simulink model "compared_sim_pizeo"  (R2022b)
settings: Solver=FixedStepAuto  StartTime=0.0  StopTime=5  FixedStep=0.001  RelTol=1e-3  EnableMultiTasking=on
settings Model: Creator=Administrator  LastModifiedBy=huheyu
settings SolverCC: AlgebraicLoopSolver=TrustRegion
settings DataIOCC: LimitDataPoints=on  SaveFormat=Array  ReturnWorkspaceOutputs=off
settings OptimizationCC: LifeSpan=inf
settings DebuggingCC: UnderspecifiedInitializationDetection=Classic  MergeDetectMultiDrivingBlocksExec=none  SolverPrmCheckMsg=warning  UnconnectedInputMsg=warning  UnconnectedOutputMsg=warning  UnconnectedLineMsg=warning  StateNameClashWarn=warning  SFUnexpectedBacktrackingDiag=warning  SFNoUnconditionalDefaultTransitionDiag=warning  SFExecutionAtInitializationDiag=none  ArithmeticOperatorsInVariantConditions=warning
settings HardwareCC: ProdBitPerPointer=32  ProdBitPerSizeT=32  ProdBitPerPtrDiffT=32  ProdLargestAtomicFloat=None  ProdIntDivRoundTo=Undefined  ProdEndianess=Unspecified  ProdWordSize=32  ProdHWDeviceType=32-bit Generic
settings ModelReferenceCC: EnableRefExpFcnMdlSchedulingChecks=on  PropagateSignalLabelsOutOfModel=off
settings SFSimCC: SimUseLocalCustomCode=off  CustomCodeUndefinedFunction=UseInterfaceOnly
settings RTWCC: RTWUseLocalCustomCode=off  DLArmComputeVersion=19.05
settings CodeAppCC: StateflowObjectComments=on
settings GRTTargetCC: TargetLangStandard=C89/C90 (ANSI)
settings ConfigComp: CovMetricSettings=dw  CovSaveCumulativeToWorkspaceVar=on  CovSaveSingleToWorkspaceVar=on  CovExternalEMLEnable=off

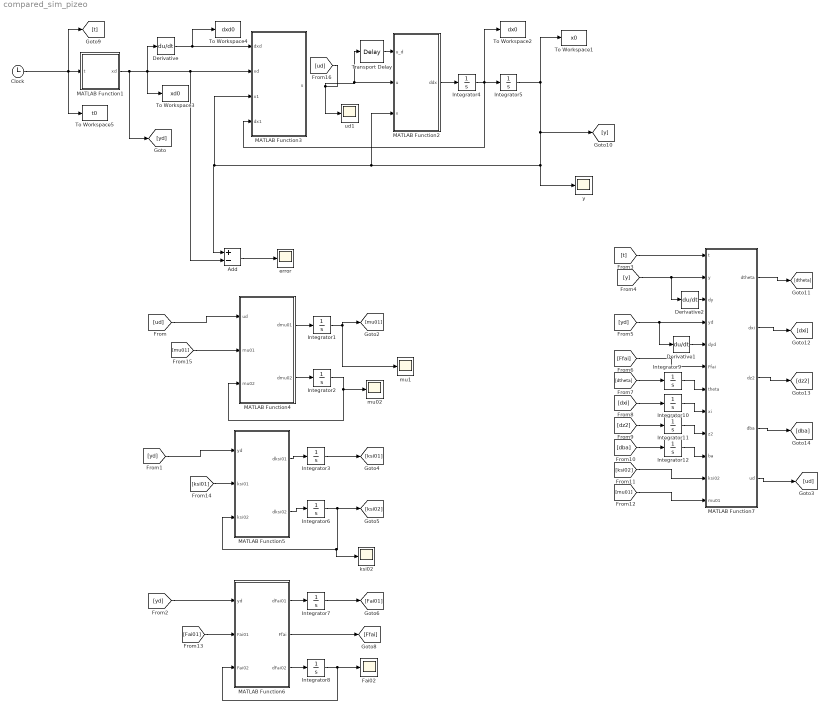
== system compared_sim_pizeo ==
  Add : Sum  Inputs=+-
  Clock : Clock
  Derivative : Derivative
  Derivative1 : Derivative
  Derivative2 : Derivative
  Fai02 : Scope
  Integrator{1..4,6..12} (11 alike) : Integrator
  Integrator5 : Integrator  InitialCondition=0.1
  MATLAB Function1 : MATLAB Function  TreatAsAtomicUnit=on
  MATLAB Function2 : MATLAB Function  TreatAsAtomicUnit=on
  MATLAB Function3 : MATLAB Function  TreatAsAtomicUnit=on
  MATLAB Function4 : MATLAB Function  TreatAsAtomicUnit=on
  MATLAB Function5 : MATLAB Function  TreatAsAtomicUnit=on
  MATLAB Function6 : MATLAB Function  TreatAsAtomicUnit=on
  MATLAB Function7 : MATLAB Function  TreatAsAtomicUnit=on
  To Workspace1 : ToWorkspace  VariableName=x0  SampleTime=-1
  To Workspace2 : ToWorkspace  VariableName=dx0  SampleTime=-1
  To Workspace3 : ToWorkspace  VariableName=xd0  SampleTime=-1
  To Workspace4 : ToWorkspace  VariableName=dxd0  SampleTime=-1
  To Workspace5 : ToWorkspace  VariableName=t0  SampleTime=-1
  Transport Delay : TransportDelay  DelayTime=0.001
  error : Scope
  ksi02 : Scope
  mu02 : Scope
  mu1 : Scope
  ud1 : Scope
  y : Scope
  wires:
  Clock/1 -> [t], To Workspace5/1, MATLAB Function1/1(t)
  MATLAB Function1/1(xd) -> [yd], Derivative/1, Add/2, MATLAB Function3/2(xd), To Workspace3/1
  Integrator5/1 -> To Workspace1/1, [y], y/1, MATLAB Function3/3(x1), Add/1, MATLAB Function2/3(x)
  Derivative/1 -> To Workspace4/1, MATLAB Function3/1(dxd)
  MATLAB Function2/1(ddx) -> Integrator4/1
  [ud] -> Transport Delay/1, MATLAB Function2/2(u), ud1/1
  Add/1 -> error/1
  Transport Delay/1 -> MATLAB Function2/1(u_d)
  Integrator4/1 -> MATLAB Function3/4(dx1), To Workspace2/1, Integrator5/1
  [ud] -> MATLAB Function4/1(ud)
  MATLAB Function4/1(dmu01) -> Integrator1/1
  MATLAB Function4/2(dmu02) -> Integrator2/1
  Integrator2/1 -> mu02/1, MATLAB Function4/3(mu02)
  MATLAB Function5/1(dksi01) -> Integrator3/1
  MATLAB Function5/2(dksi02) -> Integrator6/1
  Integrator6/1 -> [ksi02], ksi02/1, MATLAB Function5/3(ksi02)
  [yd] -> MATLAB Function5/1(yd)
  Integrator8/1 -> Fai02/1, MATLAB Function6/3(Fai02)
  MATLAB Function6/3(dFai02) -> Integrator8/1
  MATLAB Function6/1(dFai01) -> Integrator7/1
  [yd] -> MATLAB Function6/1(yd)
  Integrator3/1 -> [ksi01]
  Integrator7/1 -> [Fai01]
  MATLAB Function6/2(Ffai) -> [Ffai]
  [t] -> MATLAB Function7/1(t)
  [y] -> Derivative2/1, MATLAB Function7/2(y)
  [yd] -> Derivative1/1, MATLAB Function7/4(yd)
  Derivative1/1 -> MATLAB Function7/5(dyd)
  [Ffai] -> MATLAB Function7/6(Ffai)
  MATLAB Function7/1(dtheta) -> [dtheta]
  [dtheta] -> Integrator9/1
  MATLAB Function7/2(dxi) -> [dxi]
  MATLAB Function7/3(dz2) -> [dz2]
  MATLAB Function7/4(dba) -> [dba]
  [dxi] -> Integrator10/1
  [dz2] -> Integrator11/1
  [dba] -> Integrator12/1
  [ksi02] -> MATLAB Function7/11(ksi02)
  [mu01] -> MATLAB Function7/12(mu01)
  Integrator9/1 -> MATLAB Function7/7(theta)
  Integrator10/1 -> MATLAB Function7/8(xi)
  Integrator11/1 -> MATLAB Function7/9(z2)
  Integrator12/1 -> MATLAB Function7/10(ba)
  [Fai01] -> MATLAB Function6/2(Fai01)
  [ksi01] -> MATLAB Function5/2(ksi01)
  [mu01] -> MATLAB Function4/2(mu01)
  MATLAB Function7/5(ud) -> [ud]
  Integrator1/1 -> [mu01], mu1/1
  Derivative2/1 -> MATLAB Function7/3(dy)

== matlab function compared_sim_pizeo/MATLAB Function6 ==
  data: yd input; Fai01 input; Fai02 input; dFai01 output; Ffai output; dFai02 output
function [dFai01,Ffai,dFai02] = getxx(yd,Fai01,Fai02)

k=6; q1=3;q2=2;
fai1=exp(-(yd-0)*(yd-0)/4);
fai2=exp(-(yd-0)*(yd-0)/8);

dFai01=-k*q1*Fai01+k*Fai02+0.1*fai1;
dFai02=-k*q2*Fai01+0.001*1/k*fai2;
Ffai=fai1+k*Fai02;

== matlab function compared_sim_pizeo/MATLAB Function7 ==
  data: t input; y input; dy input; yd input; dtheta output; dxi output; dyd input; Ffai input; theta input; xi input; z2 input; ba input; dz2 output; dba output; ud output; ksi02 input; mu01 input
function [dtheta,dxi,dz2,dba,ud] = getxx(t,y,dy,yd,dyd,Ffai,theta,xi,z2,ba,ksi02,mu01)
k=6; l1=0.030; l2=0.040;
KK2=0.05;q2=2;
gama_theta=10;
gama_xi=8;sigma_xi=0.06;
gama_b=9;sigma_b=0.06;
et=y-yd;
pt=1*exp(-3*t)+0.5;
S1=tan(pi*et/(2*pt));
dtheta=gama_theta*(theta*S1*Ffai*Ffai-sigma_b*theta);
pbmu02=(-l1*S1-k*ksi02-theta*S1*Ffai*Ffai+dyd)/k;
dxi=-gama_xi*(k*pbmu02*S1+sigma_xi*xi);
bmu02=dxi*pbmu02;
dz2=(bmu02-z2)/KK2;
S2=bmu02-z2;
dba=gama_b*(k*S1*S2-sigma_b*ba);
ud=-100*ba*S1+dz2-l2*S2-300*(dy-dyd);

== matlab function compared_sim_pizeo/MATLAB Function1 ==
  data: t input; xd output
function xd= getxx(t)
xd=sin(2*pi*t);

== matlab function compared_sim_pizeo/MATLAB Function3 ==
  data: dxd input; u output; xd input; x1 input; dx1 input
%function [u,dtheta1_hat,dtheta2_hat]= getxx(t,dxd,xd,x1,dx1,theta1_hat,theta2_hat)
function u = getxx(dxd,xd,x1,dx1)

%T=1; epison=1;
k1=30;k2=100;
%r1=0.5;r2=0.1;

%if t<T
%    Yeta1=(1/(t+0.01)-1/T)^3+epison;
%    if Yeta1>10
%        Yeta1=100;
%    end
%else
%    Yeta1=epison;
%end
%e=x1-xd;
%h11=1-(e/Yeta1)^2;


%F1=30;F2=500;
%h12=1-(x1/F1)^2;
%h2=1-(dx1/F2)^2;
%h1=h11*h12/(h11+h12);


%ksi1=e/h1;
%ksi2=dx1/h2;
%mu1=1/h1;
%mu2=1/h2;

%z1=ksi1;
%ci1=[0 0 0 0]';
%xi1=[x1,xd,dx1,dxd]';

%fai1=exp(-(xi1-ci1)'*(xi1-ci1)/4);
%faic1=fai1*fai1+1;

%alpha1=1/h2*(-k1*z1+dxd-r1*mu1*theta1_hat*faic1*z1);
%dtheta1_hat=-r1*theta1_hat+r1*mu1*mu1*faic1*z1*z1;

%ci2=[0 0 0 0]';
%xi2=[x1,xd,dx1,dxd]';
%fai2=exp(-(xi2-ci2)'*(xi2-ci2)/4);
%faic2=fai2*fai2+1;

%z2=ksi2-alpha1;
%dtheta2_hat=-r2*theta2_hat+r2*mu2*mu2*z2*z2*faic2;
%u=-k2*z2-0*1/mu2*mu1*mu1*h2*h2*z1*z1*z2-r2*mu2*theta2_hat*faic1*z2;

u=-k1*(x1-xd)-k2*(dx1-dxd);

== matlab function compared_sim_pizeo/MATLAB Function2 ==
  data: u_d input; u input; ddx output; x input
function ddx= getxx(u_d,u,x)



   r=0.6;
   rho=10*tanh(u);
   fr=max(rho-r,min(rho+r,u_d));
   pr=0.6*exp(-0.108*(r-0.5)^2);
   w1=0.45*u+fr*pr;
   w=double(w1);

ddx=-0.5*sin(x)+0.01*cos(5*x)+w;

== matlab function compared_sim_pizeo/MATLAB Function4 ==
  data: ud input; mu01 input; mu02 input; dmu01 output; dmu02 output
function [dmu01,dmu02] = getxx(ud,mu01,mu02)

k=6;q1=3;q2=2;

dmu01=-100*k*q1*mu01+1*k*mu02;
dmu02=-100*k*q2*mu01+1/k*ud;

== matlab function compared_sim_pizeo/MATLAB Function5 ==
  data: yd input; ksi01 input; ksi02 input; dksi01 output; dksi02 output
function [dksi01,dksi02] = getxx(yd,ksi01,ksi02)

k=6; q1=3;q2=2;

dksi01=-k*q1*ksi01+k*ksi02+k*q1*yd;
dksi02=-k*q2*ksi01+k*q2*yd;
